simulink model "k1visey"  (Simulink 8.5)
settings: Solver=ode45  StartTime=0.0  StopTime=10.0  RelTol=1e-3
libraries: cdsCDI64 x2, cdsCDO64 x2, dac x2, cdsAdcx0 x1, cdsAdcx1 x1, TYPEA_MASTER x1, cdsParameters x1
settings Model: Creator=controls  LastModifiedBy=controls
settings DataIOCC: SignalLoggingSaveFormat=Dataset
settings OptimizationCC: ExpressionDepthLimit=128
settings DebuggingCC: UnderspecifiedInitializationDetection=Simplified  MergeDetectMultiDrivingBlocksExec=error  FcnCallInpInsideContextMsg=EnableAllAsError  StateNameClashWarn=none
settings GRTTargetCC: CombineOutputUpdateFcns=on  GRTInterface=off

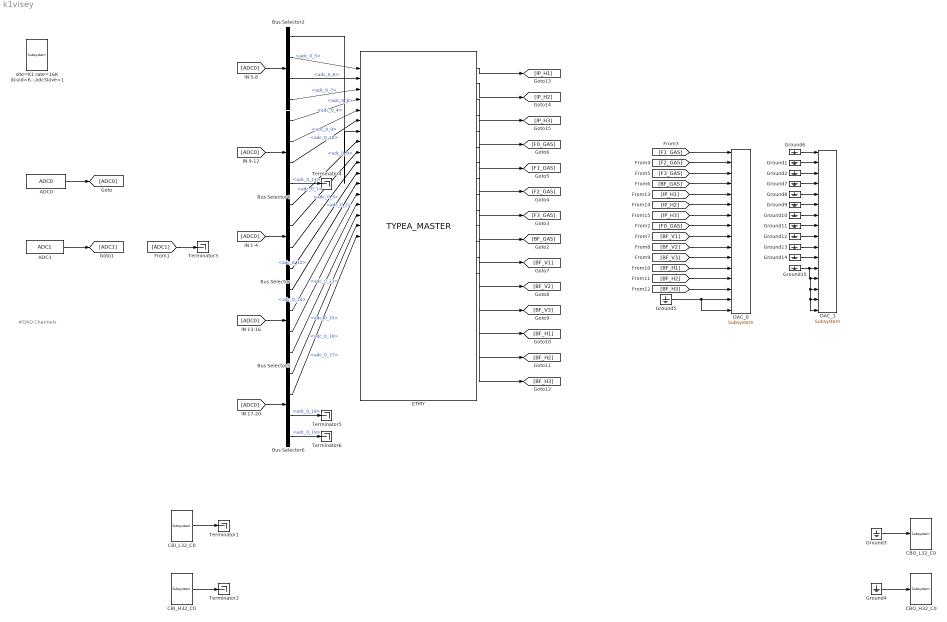
== system k1visey ==
  note: #DAQ Channels
  ADC0 : cdsAdcx0/ADC0  Tag=cdsAdc  Description=|
      | type-GSC_16AI64SSA
      | card_num=0
      settings: AttributesFormatString=%<Description>\n%<Tag>
  ADC1 : cdsAdcx1/ADC1  Tag=cdsAdc  Description=|
      | type-GSC_16AI64SSA
      | card_num=1
      settings: AttributesFormatString=%<Description>\n%<Tag>
  Bus Selector : BusSelector  OutputSignals=adc_0_0,adc_0_1,adc_0_2,adc_0_3
  Bus Selector2 : BusSelector  OutputSignals=adc_0_4,adc_0_5,adc_0_6,adc_0_7
  Bus Selector4 : BusSelector  OutputSignals=adc_0_8,adc_0_9,adc_0_10,adc_0_11
  Bus Selector5 : BusSelector  OutputSignals=adc_0_12,adc_0_13,adc_0_14,adc_0_15
  Bus Selector6 : BusSelector  OutputSignals=adc_0_16,adc_0_17,adc_0_18,adc_0_19
  CBI_H32_C0 : cdsCDI64/Subsystem  Tag=cdsCDI64  Description=card_num=1
      settings: AttributesFormatString=%<Tag>\n%<Description>
  CBI_L32_C0 : cdsCDI64/Subsystem  Tag=cdsCDI64  Description=card_num=0
      settings: AttributesFormatString=%<Tag>\n%<Description>
  CBO_H32_C0 : cdsCDO64/Subsystem  Tag=cdsCDO64  Description=card_num=1
      settings: AttributesFormatString=%<Tag>\n%<Description>
  CBO_L32_C0 : cdsCDO64/Subsystem  Tag=cdsCDO64  Description=card_num=0
      settings: AttributesFormatString=%<Tag>\n%<Description>
  DAC_0 : dac/Subsystem  Description=|
      | type=GSC_16AO16,
      | card_num=0
      settings: AttributesFormatString=%<Description>
  DAC_1 : dac/Subsystem  Description=|
      | type=GSC_16AO16,
      | card_num=1
      settings: AttributesFormatString=%<Description>
  ETMY : TYPEA_MASTER/TYPEA_MASTER
  Ground{1..15} (15 alike) : Ground
  Terminator{1..6} (6 alike) : Terminator
  site=K1 rate=16K dcuid=666 host=k1ey1 specific_cpu=3 adcSlave=1 : cdsParameters/Subsystem  Tag=cdsParameters  Description=|
      | Purpose:                                                                                                                                                                                                                                
      | Provide system parameters to the FE code generator to properly configure the generated EPICS names, rep rate of the FE controller, and the Data Acquisition node ID for proper storage of data from this FE controller.                 
      |                                                                                                                                                                                                                                         
      | Useage:                                                                                                                                                                                                                                 
      | The part NAME field is used to identify the FE parameters. It must be of the form:                                                                                                                                                      
      | site=                                                                                                                                                                                                                                   
      | rate=                                                                                                                                                                                                                                   
      | dcuid=                                                                                                                                                                                                                                  
      |                                                                                                                                                                                                                                         
      | Where:                                                                                                                                                                                                                                  
      | site= argument may be H1, H2, L1, M1, G1, either as a single argument or multiple, for example site=H1,H2. These are the only names allowed. These will become the first two characters of all EPICS and signal names (for example G1:).
      |                                                                                                                                                                                                                                         
      | rate= may be 2K, 16K, 32K, or 64K                                                                                                                                                                                                       
      |                                                                                                                                                                                                                                         
      | dcuid= is site specific ie it must be unique at each site.
      settings: AttributesFormatString=%<Tag>
  wires:
  ADC0/1 -> [ADC0]
  ADC1/1 -> [ADC1]
  ETMY/4 -> [F0_GAS]
  ETMY/5 -> [F1_GAS]
  ETMY/8 -> [BF_GAS]
  ETMY/7 -> [F3_GAS]
  ETMY/6 -> [F2_GAS]
  [BF_GAS] -> DAC_0/4
  [F3_GAS] -> DAC_0/3
  [F2_GAS] -> DAC_0/2
  [F1_GAS] -> DAC_0/1
  [ADC0] -> Bus Selector/1
  Bus Selector/4 -> ETMY/11  "<adc_0_3>"
  Bus Selector/3 -> ETMY/10  "<adc_0_2>"
  Bus Selector/2 -> ETMY/9  "<adc_0_1>"
  Bus Selector/1 -> ETMY/8  "<adc_0_0>"
  [F0_GAS] -> DAC_0/8
  [ADC1] -> Terminator3/1
  Ground5/1 -> DAC_0/16, DAC_0/15
  Ground14/1 -> DAC_1/11
  Ground1/1 -> DAC_1/2
  Ground13/1 -> DAC_1/10
  Ground9/1 -> DAC_1/6
  Ground2/1 -> DAC_1/3
  Ground7/1 -> DAC_1/4
  Ground6/1 -> DAC_1/1
  Ground10/1 -> DAC_1/7
  Ground8/1 -> DAC_1/5
  Ground11/1 -> DAC_1/8
  Ground12/1 -> DAC_1/9
  [ADC0] -> Bus Selector2/1
  Bus Selector2/2 -> ETMY/1  "<adc_0_5>"
  Bus Selector2/3 -> ETMY/2  "<adc_0_6>"
  Bus Selector2/4 -> ETMY/3  "<adc_0_7>"
  Bus Selector2/1 -> ETMY/7  "<adc_0_4>"
  [ADC0] -> Bus Selector4/1
  Bus Selector4/1 -> ETMY/4  "<adc_0_8>"
  Bus Selector4/2 -> ETMY/5  "<adc_0_9>"
  Bus Selector4/3 -> ETMY/6  "<adc_0_10>"
  Bus Selector4/4 -> Terminator4/1  "<adc_0_11>"
  [ADC0] -> Bus Selector5/1
  Bus Selector5/4 -> ETMY/15  "<adc_0_15>"
  Bus Selector5/1 -> ETMY/12  "<adc_0_12>"
  Bus Selector5/3 -> ETMY/14  "<adc_0_14>"
  Bus Selector5/2 -> ETMY/13  "<adc_0_13>"
  [ADC0] -> Bus Selector6/1
  Bus Selector6/1 -> ETMY/16  "<adc_0_16>"
  Bus Selector6/2 -> ETMY/17  "<adc_0_17>"
  Bus Selector6/3 -> Terminator5/1  "<adc_0_18>"
  Bus Selector6/4 -> Terminator6/1  "<adc_0_19>"
  ETMY/9 -> [BF_V1]
  Ground15/1 -> DAC_1/16, DAC_1/15, DAC_1/14, DAC_1/13, DAC_1/12
  ETMY/10 -> [BF_V2]
  ETMY/11 -> [BF_V3]
  ETMY/12 -> [BF_H1]
  ETMY/13 -> [BF_H2]
  ETMY/14 -> [BF_H3]
  [BF_H2] -> DAC_0/13
  [BF_V3] -> DAC_0/11
  [BF_H3] -> DAC_0/14
  [BF_V1] -> DAC_0/9
  [BF_H1] -> DAC_0/12
  [BF_V2] -> DAC_0/10
  ETMY/1 -> [IP_H1]
  ETMY/2 -> [IP_H2]
  ETMY/3 -> [IP_H3]
  [IP_H2] -> DAC_0/6
  [IP_H3] -> DAC_0/7
  [IP_H1] -> DAC_0/5
  CBI_L32_C0/1 -> Terminator1/1
  CBI_H32_C0/1 -> Terminator2/1
  Ground3/1 -> CBO_L32_C0/1
  Ground4/1 -> CBO_H32_C0/1
